simulink model "ben2asys"  (Simulink 6.0)
settings: Solver=ode15s  SolverMode=SingleTasking  StartTime=0.0  StopTime=5  RelTol=1e-3  AbsTol=1e-6
PreLoadFcn:
  | ben2adat
values from neighbouring files (symbols this model uses):
  a1 = 0.08197    [ben2adat.m]    (also in ben2bdat.m; ben2cdat.m)
  a11 = 0.3077    [ben2adat.m]    (also in ben2bdat.m; ben2cdat.m)
  a12 = 3.2314    [ben2adat.m]    (also in ben2bdat.m; ben2cdat.m)
  a13 = 0.8597    [ben2adat.m]    (also in ben2bdat.m; ben2cdat.m)
  a14 = -0.002323    [ben2adat.m]    (also in ben2bdat.m; ben2cdat.m)
  a15 = -0.01139    [ben2adat.m]    (also in ben2bdat.m; ben2cdat.m)
  a16 = 45.112    [ben2adat.m]    (also in ben2bdat.m; ben2cdat.m)
  a5 = 0.2551    [ben2adat.m]    (also in ben2bdat.m; ben2cdat.m)
  a8 = -0.4283    [ben2adat.m]    (also in ben2bdat.m; ben2cdat.m)
  a9 = 0.6645    [ben2adat.m]    (also in ben2bdat.m; ben2cdat.m)
  gd2 = [1/220,1]    [ben2adat.m]    (also in ben2bdat.m; ben2cdat.m; ben3adat.m = [1,6,13]; ben3bdat.m = [1,6,13])
  gd3 = [1/85/85,1.2/85,1]    [ben2adat.m]    (also in ben2bdat.m; ben2cdat.m; ben3adat.m = [1,-1]; ben3bdat.m = [1,-1])
  gd5 = [1/170,1]    [ben2adat.m]    (also in ben2bdat.m; ben2cdat.m; ben3adat.m = [1,-1]; ben3bdat.m = [1,-1])
  gd61 = [1/80,1]    [ben2adat.m]    (also in ben2bdat.m; ben2cdat.m)
  gd62 = [1/160/160,0.6/160,1]    [ben2adat.m]    (also in ben2bdat.m; ben2cdat.m)
  gd63 = [1/1600,1]    [ben2adat.m]    (also in ben2bdat.m; ben2cdat.m)
  gd7 = [1,0]    [ben2adat.m]    (also in ben2bdat.m; ben2cdat.m; ben3adat.m = [1,-0.9277]; ben3bdat.m = [1,-0.9277])
  gd91 = [1,0]    [ben2adat.m]    (also in ben2bdat.m; ben2cdat.m; ben3bdat.m = [1,.25*200,200*200])
  gd92 = [1/50,1]    [ben2adat.m]    (also in ben2bdat.m; ben2cdat.m; ben3bdat.m = [1,0])
  gn2 = 1    [ben2adat.m]    (also in ben2bdat.m; ben2cdat.m; ben3adat.m = [-0.1,9]; ben3bdat.m = [-0.1,9])
  gn3 = 1    [ben2adat.m]    (also in ben2bdat.m; ben2cdat.m; ben3adat.m = .2625*[1,-0.9048]; ben3bdat.m = .2625*[1,-0.9048])
  gn5 = 1    [ben2adat.m]    (also in ben2bdat.m; ben2cdat.m; ben3adat.m = 1.035*[1,-0.9324]; ben3bdat.m = 1.035*[1,-0.9324])
  gn61 = [1,0]    [ben2adat.m]    (also in ben2bdat.m; ben2cdat.m)
  gn62 = [1/30,1]    [ben2adat.m]    (also in ben2bdat.m; ben2cdat.m)
  gn63 = 1    [ben2adat.m]    (also in ben2bdat.m; ben2cdat.m)
  gn7 = 1    [ben2adat.m]    (also in ben2bdat.m; ben2cdat.m; ben3adat.m = 0.0362*[1,1]; ben3bdat.m = 0.0362*[1,1])
  gn91 = [1,1.5]    [ben2adat.m]    (also in ben2bdat.m; ben2cdat.m; ben3bdat.m = 40000)
  gn92 = [1/150,1]    [ben2adat.m]    (also in ben2bdat.m; ben2cdat.m; ben3bdat.m = 1)
  k1 = 1    [ben2adat.m]    (also in ben2bdat.m; ben2cdat.m)
  k2 = 1.25    [ben2adat.m]    (also in ben2bdat.m; ben2cdat.m)
  k3 = 0.001244    [ben2adat.m]    (also in ben2bdat.m; ben2cdat.m)
  k4 = 0.1    [ben2adat.m]    (also in ben2bdat.m; ben2cdat.m)
  k5 = 0.01125    [ben2adat.m]    (also in ben2bdat.m; ben2cdat.m)
  k6 = 0.06    [ben2adat.m]    (also in ben2bdat.m; ben2cdat.m)
  k9 = 29.82    [ben2adat.m]    (also in ben2bdat.m; ben2cdat.m)
settings Model: Creator=The MathWorks Inc.  LastModifiedBy=batserve  ExtModeTrigMode=oneshot  ExtModeArmWhenConnect=off  ExtModeAutoUpdateStatusClock=off
settings DataIOCC: ExternalInput=[]  InitialState=[]  LimitDataPoints=off  SaveOutput=off  SaveTime=off
settings OptimizationCC: BooleanDataType=off
settings DebuggingCC: CheckExecutionContextPreStartOutputMsg=on  CheckExecutionContextRuntimeOutputMsg=on  SolverPrmCheckMsg=none  IntegerOverflowMsg=none
settings HardwareCC: TargetUnknown=on

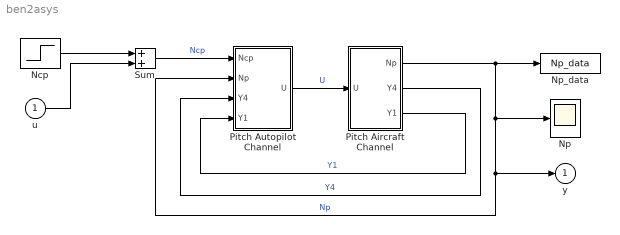
== system ben2asys ==
  u : Inport  Port=1  LatchInput=off
  Ncp : Step  Time=0  SampleTime=0
  Np : Scope
      settings: TickLabels=on  TimeRange=5  YMin=-0.2  YMax=1.4  DataFormat=Array
  Np_data : ToWorkspace  VariableName=Np_data  SampleTime=-1  SaveFormat=Array
  Pitch Aircraft Channel : Subsystem  PropExecContextAcrossSSBoundary=on
  Pitch Autopilot Channel : Subsystem  PropExecContextAcrossSSBoundary=on
  Sum : Sum  SaturateOnIntegerOverflow=on  InputSameDT=on
  y : Outport  InitialOutput=0
  wires:
  u/1 -> Sum/2
  Ncp/1 -> Sum/1
  Sum/1 -> Pitch Autopilot Channel/1(Ncp)  "Ncp"
  Pitch Aircraft Channel/1(Np) -> Np/1, Pitch Autopilot Channel/2(Np), y/1, Np_data/1  "Np"
  Pitch Aircraft Channel/2(Y4) -> Pitch Autopilot Channel/3(Y4)  "Y4"
  Pitch Aircraft Channel/3(Y1) -> Pitch Autopilot Channel/4(Y1)  "Y1"
  Pitch Autopilot Channel/1(U) -> Pitch Aircraft Channel/1(U)  "U"

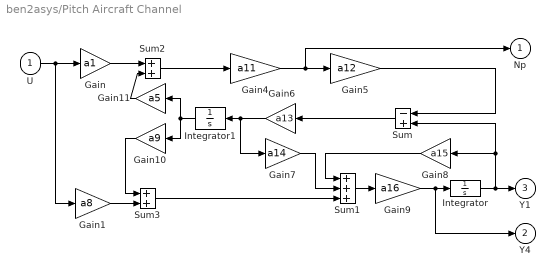
== system ben2asys/Pitch Aircraft Channel ==
  U : Inport  Port=1  LatchInput=off
  Gain : Gain  Gain=a1  SaturateOnIntegerOverflow=on
  Gain1 : Gain  Gain=a8  SaturateOnIntegerOverflow=on
  Gain10 : Gain  Orientation=left  Gain=a9  SaturateOnIntegerOverflow=on
  Gain11 : Gain  Orientation=left  Gain=a5  SaturateOnIntegerOverflow=on
  Gain4 : Gain  Gain=a11  SaturateOnIntegerOverflow=on
  Gain5 : Gain  Gain=a12  SaturateOnIntegerOverflow=on
  Gain6 : Gain  Orientation=left  Gain=a13  SaturateOnIntegerOverflow=on
  Gain7 : Gain  Gain=a14  SaturateOnIntegerOverflow=on
  Gain8 : Gain  Orientation=left  Gain=a15  SaturateOnIntegerOverflow=on
  Gain9 : Gain  Gain=a16  SaturateOnIntegerOverflow=on
  Integrator : Integrator
  Integrator1 : Integrator  Orientation=left
  Sum : Sum  Orientation=left  Inputs=-+  SaturateOnIntegerOverflow=on  InputSameDT=on
  Sum1 : Sum  Inputs=3  SaturateOnIntegerOverflow=on  InputSameDT=on
  Sum2 : Sum  Inputs=2  SaturateOnIntegerOverflow=on  InputSameDT=on
  Sum3 : Sum  Inputs=2  SaturateOnIntegerOverflow=on  InputSameDT=on
  Np : Outport  InitialOutput=0
  Y4 : Outport  Port=2  InitialOutput=0
  Y1 : Outport  Port=3  InitialOutput=0
  wires:
  Integrator1/1 -> Gain10/1, Gain11/1
  Gain/1 -> Sum2/1
  Gain11/1 -> Sum2/2
  Gain1/1 -> Sum3/2
  Gain10/1 -> Sum3/1
  Sum2/1 -> Gain4/1
  Sum3/1 -> Sum1/3
  Sum1/1 -> Gain9/1
  Gain8/1 -> Sum1/1
  Gain5/1 -> Sum/1
  Sum/1 -> Gain6/1
  Integrator/1 -> Y1/1, Sum/2, Gain8/1
  Gain9/1 -> Integrator/1, Y4/1
  U/1 -> Gain/1, Gain1/1
  Gain7/1 -> Sum1/2
  Gain6/1 -> Integrator1/1, Gain7/1
  Gain4/1 -> Gain5/1, Np/1

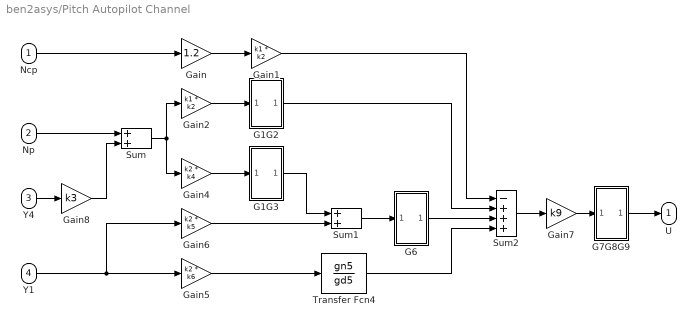
== system ben2asys/Pitch Autopilot Channel ==
  Ncp : Inport  Port=1  LatchInput=off
  Np : Inport  Port=2  LatchInput=off
  Y4 : Inport  Port=3  LatchInput=off
  Y1 : Inport  Port=4  LatchInput=off
  G1G2 : Subsystem  PropExecContextAcrossSSBoundary=on
  G1G3 : Subsystem  PropExecContextAcrossSSBoundary=on
  G6 : Subsystem  PropExecContextAcrossSSBoundary=on
  G7G8G9 : Subsystem  PropExecContextAcrossSSBoundary=on
  Gain : Gain  Gain=1.2  SaturateOnIntegerOverflow=on
  Gain1 : Gain  Gain=k1 * k2  SaturateOnIntegerOverflow=on
  Gain2 : Gain  Gain=k1 * k2  SaturateOnIntegerOverflow=on
  Gain4 : Gain  Gain=k2 * k4  SaturateOnIntegerOverflow=on
  Gain5 : Gain  Gain=k2 * k6  SaturateOnIntegerOverflow=on
  Gain6 : Gain  Gain=k2 * k5  SaturateOnIntegerOverflow=on
  Gain7 : Gain  Gain=k9  SaturateOnIntegerOverflow=on
  Gain8 : Gain  Gain=k3  SaturateOnIntegerOverflow=on
  Sum : Sum  Inputs=2  SaturateOnIntegerOverflow=on  InputSameDT=on
  Sum1 : Sum  Inputs=2  SaturateOnIntegerOverflow=on  InputSameDT=on
  Sum2 : Sum  Inputs=-+++  SaturateOnIntegerOverflow=on  InputSameDT=on
  Transfer Fcn4 : TransferFcn  Numerator=gn5  Denominator=gd5
  U : Outport  InitialOutput=0
  wires:
  Sum/1 -> Gain2/1, Gain4/1
  Y1/1 -> Gain5/1, Gain6/1
  Sum1/1 -> G6/1(In)
  Gain7/1 -> G7G8G9/1(In)
  Sum2/1 -> Gain7/1
  Gain/1 -> Gain1/1
  Y4/1 -> Gain8/1
  Np/1 -> Sum/1
  Ncp/1 -> Gain/1
  G1G3/1(Out) -> Sum1/1
  Gain4/1 -> G1G3/1(In)
  Gain2/1 -> G1G2/1(In)
  Gain5/1 -> Transfer Fcn4/1
  Gain6/1 -> Sum1/2
  Transfer Fcn4/1 -> Sum2/4
  G6/1(Out) -> Sum2/3
  Gain8/1 -> Sum/2
  Gain1/1 -> Sum2/1
  G1G2/1(Out) -> Sum2/2
  G7G8G9/1(Out) -> U/1

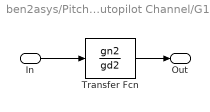
== system ben2asys/Pitch Autopilot Channel/G1G2 ==
  In : Inport  Port=1  LatchInput=off
  Transfer Fcn : TransferFcn  Numerator=gn2  Denominator=gd2
  Out : Outport  InitialOutput=0
  wires:
  In/1 -> Transfer Fcn/1
  Transfer Fcn/1 -> Out/1

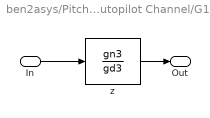
== system ben2asys/Pitch Autopilot Channel/G1G3 ==
  In : Inport  Port=1  LatchInput=off
  z : TransferFcn  Numerator=gn3  Denominator=gd3
  Out : Outport  InitialOutput=0
  wires:
  In/1 -> z/1
  z/1 -> Out/1

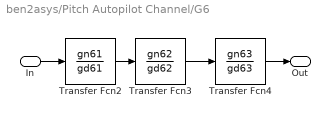
== system ben2asys/Pitch Autopilot Channel/G6 ==
  In : Inport  Port=1  LatchInput=off
  Transfer Fcn2 : TransferFcn  Numerator=gn61  Denominator=gd61
  Transfer Fcn3 : TransferFcn  Numerator=gn62  Denominator=gd62
  Transfer Fcn4 : TransferFcn  Numerator=gn63  Denominator=gd63
  Out : Outport  InitialOutput=0
  wires:
  In/1 -> Transfer Fcn2/1
  Transfer Fcn2/1 -> Transfer Fcn3/1
  Transfer Fcn3/1 -> Transfer Fcn4/1
  Transfer Fcn4/1 -> Out/1

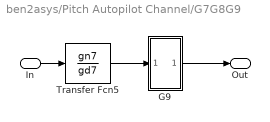
== system ben2asys/Pitch Autopilot Channel/G7G8G9 ==
  In : Inport  Port=1  LatchInput=off
  G9 : Subsystem  PropExecContextAcrossSSBoundary=on
  Transfer Fcn5 : TransferFcn  Numerator=gn7  Denominator=gd7
  Out : Outport  InitialOutput=0
  wires:
  In/1 -> Transfer Fcn5/1
  G9/1(Out) -> Out/1
  Transfer Fcn5/1 -> G9/1(In)

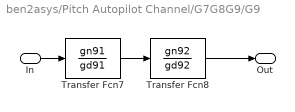
== system ben2asys/Pitch Autopilot Channel/G7G8G9/G9 ==
  In : Inport  Port=1  LatchInput=off
  Transfer Fcn7 : TransferFcn  Numerator=gn91  Denominator=gd91
  Transfer Fcn8 : TransferFcn  Numerator=gn92  Denominator=gd92
  Out : Outport  InitialOutput=0
  wires:
  In/1 -> Transfer Fcn7/1
  Transfer Fcn7/1 -> Transfer Fcn8/1
  Transfer Fcn8/1 -> Out/1
